simulink model "Pendulo_doble"  (R2022b)
settings: Solver=ode4  StartTime=0  StopTime=10  FixedStep=0.0001  RelTol=1e-3
undefined symbols (not defined in the file): g, L1, L2, m1, m2
settings Model: Creator=mluser  LastModifiedBy=mluser

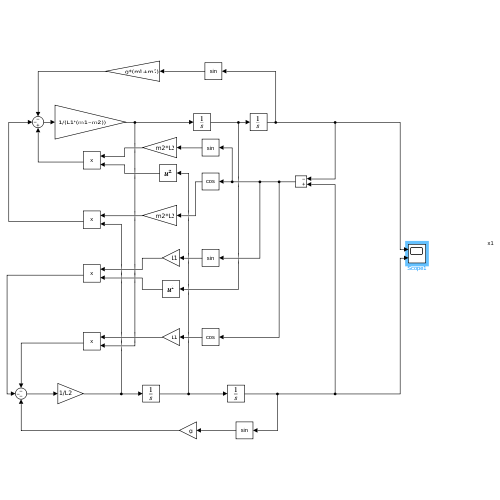
[thumbnail: Simulink's stored preview of the top-level diagram]
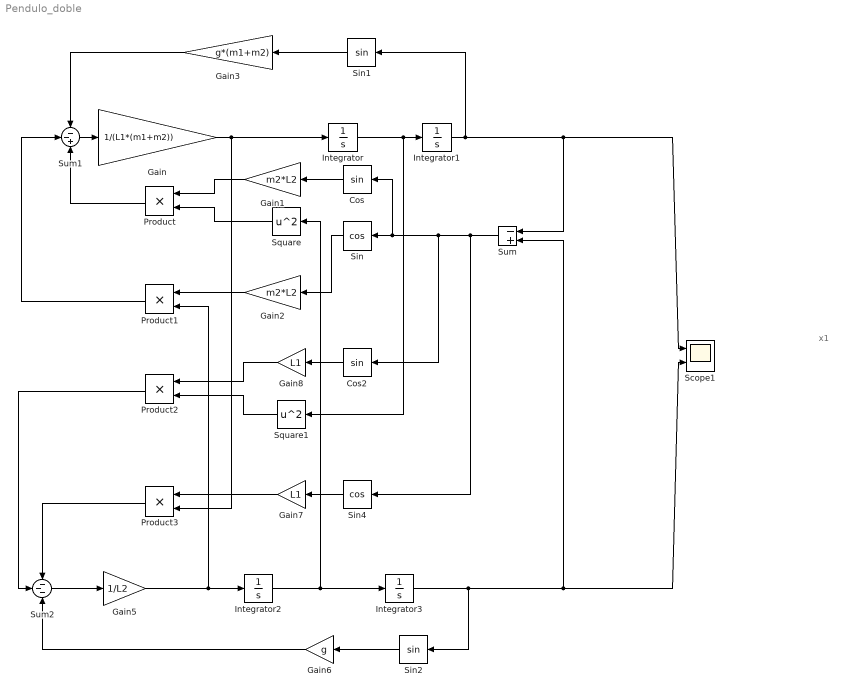
== system Pendulo_doble ==
  note: x1
  Cos : Trigonometry
  Cos2 : Trigonometry
  Gain : Gain  Gain=1/(L1*(m1+m2))
  Gain1 : Gain  Gain=m2*L2
  Gain2 : Gain  Gain=m2*L2
  Gain3 : Gain  Gain=g*(m1+m2)
  Gain5 : Gain  Gain=1/L2
  Gain6 : Gain  Gain=g
  Gain7 : Gain  Gain=L1
  Gain8 : Gain  Gain=L1
  Integrator : Integrator
  Integrator1 : Integrator
  Integrator2 : Integrator
  Integrator3 : Integrator  InitialCondition=(7*pi)/36
  Product{,1..3} (4 alike) : Product
  Scope1 : Scope  NumInputPorts=2
  Sin : Trigonometry  Operator=cos
  Sin1 : Trigonometry
  Sin2 : Trigonometry
  Sin4 : Trigonometry  Operator=cos
  Square : Math  Operator=square
  Square1 : Math  Operator=square
  Sum : Sum  Inputs=-+
  Sum1 : Sum  Inputs=--+
  Sum2 : Sum  Inputs=---
  wires:
  Gain/1 -> Product3/2, Integrator/1
  Integrator/1 -> Square1/1, Integrator1/1
  Sum1/1 -> Gain/1
  Cos/1 -> Gain1/1
  Sin/1 -> Gain2/1
  Sum/1 -> Sin4/1, Cos2/1, Cos/1, Sin/1
  Gain3/1 -> Sum1/1
  Sin1/1 -> Gain3/1
  Gain5/1 -> Product1/2, Integrator2/1
  Integrator2/1 -> Square/1, Integrator3/1
  Sin2/1 -> Gain6/1
  Gain6/1 -> Sum2/3
  Sum2/1 -> Gain5/1
  Integrator3/1 -> Sum/2, Scope1/2, Sin2/1
  Gain1/1 -> Product/1
  Gain2/1 -> Product1/1
  Square/1 -> Product/2
  Product/1 -> Sum1/3
  Product1/1 -> Sum1/2
  Cos2/1 -> Gain8/1
  Sin4/1 -> Gain7/1
  Gain8/1 -> Product2/1
  Gain7/1 -> Product3/1
  Square1/1 -> Product2/2
  Product3/1 -> Sum2/1
  Product2/1 -> Sum2/2
  Integrator1/1 -> Scope1/1, Sum/1, Sin1/1
